simulink model "simulink_ros"  (R2022b)
settings: Solver=FixedStepAuto  StartTime=0.0  StopTime=10.0  FixedStep=0.01  RelTol=1e-3
libraries: robotlib x4
settings Model: Creator=pico  LastModifiedBy=pico

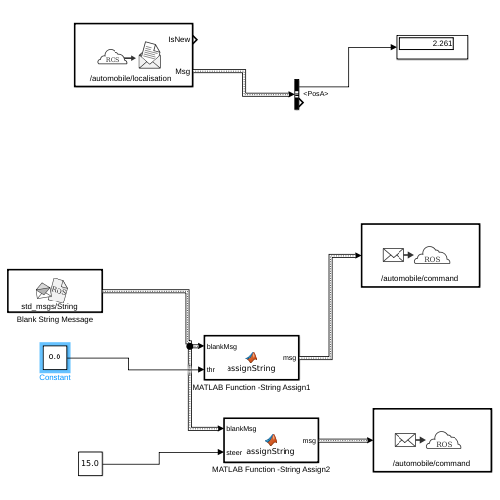
[thumbnail: Simulink's stored preview of the top-level diagram]
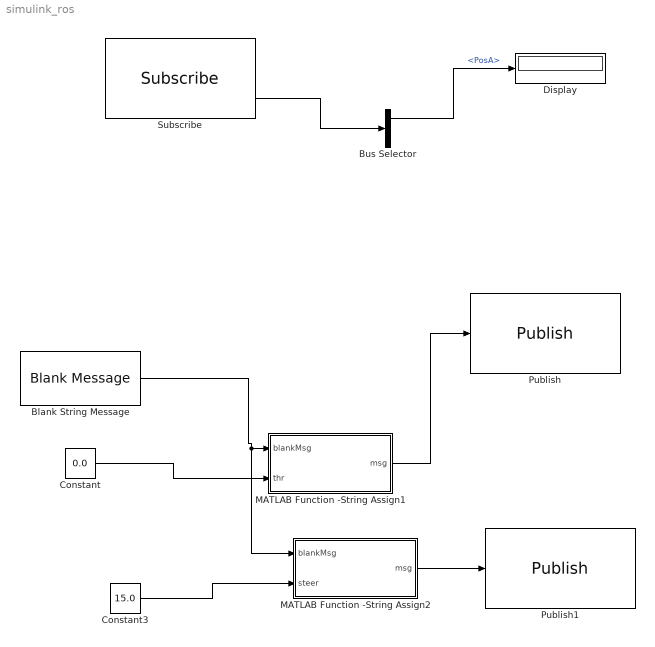
== system simulink_ros ==
  Blank String Message : robotlib/Blank Message  messageClass=Message  entityType=std_msgs/String  messageType=std_msgs/String  SampleTime=inf  legacyBusStruct=off
  Bus Selector : BusSelector  OutputSignals=PosA,PosB
  Constant : Constant  Value=0.0
  Constant3 : Constant  Value=15.0
  Display : Display
  MATLAB Function -String Assign1 : MATLAB Function  TreatAsAtomicUnit=on
  MATLAB Function -String Assign2 : MATLAB Function  TreatAsAtomicUnit=on
  Publish : robotlib/Publish  topicSource=Select from ROS network  topic=/automobile/command  messageType=std_msgs/String  legacyBusStruct=off  messageQueueLength=1
      settings: LibrarySourceBlock=roslib/ROS/Publish
  Publish1 : robotlib/Publish  topicSource=Select from ROS network  topic=/automobile/command  messageType=std_msgs/String  legacyBusStruct=off  messageQueueLength=1
      settings: LibrarySourceBlock=roslib/ROS/Publish
  Subscribe : robotlib/Subscribe  topicSource=Select from ROS network  topic=/automobile/localisation  messageType=utils/localisation  SampleTime=-1  legacyBusStruct=off  messageQueueLength=1
      settings: LibrarySourceBlock=roslib/ROS/Subscribe
  wires:
  Subscribe/2 -> Bus Selector/1
  Bus Selector/1 -> Display/1  "<PosA>"
  Blank String Message/1 -> MATLAB Function -String Assign2/1(blankMsg), MATLAB Function -String Assign1/1(blankMsg)
  MATLAB Function -String Assign1/1(msg) -> Publish/1
  Constant/1 -> MATLAB Function -String Assign1/2(thr)
  MATLAB Function -String Assign2/1(msg) -> Publish1/1
  Constant3/1 -> MATLAB Function -String Assign2/2(steer)

== matlab function simulink_ros/MATLAB Function -String Assign2 ==
  data: blankMsg input; msg output Bus: SL_Bus_simulink_ros_std_msgs_String; steer input
function msg = assignString(blankMsg,steer)
% assignString - Assign a string in a ROS message
%
% MSG = assignString(blankMsg) assigns a known string value to a 
%  string field in a ROS message, and outputs the updated ROS message.
%
%  blankMsg (input): A bus for a 'std_msgs/String' message. This is 
%      used to initialize the output. 
%  msg (output): A bus for a 'std_msgs/String' message, with the Data 
%      field set to a string.

%   Copyright 2015 The MathWorks, Inc.
%#codegen

% Note: The datatype of 'msg' has been explicitly set to the appropriate 
% Simulink bus type ("Bus: SL_Bus_robotROSMessageUsageExample_std_msgs_String"). 
%
% If the model name is changed, the datatype needs to be changed as well:
%   1) Click "Edit Data" in the Editor toolstrip to open "Ports and Data Manager"
%   2) Select "msg". From the "Type" dropdown, select "--- Refresh data types ---"
%   3) Set datatype to "Bus: SL_Bus_<modelname>_std_msgs_String"
    
% stringToAssign = 'information';
steer_string = sprintf('%.1f',steer);
% "{\"action\": \"1\", \"speed\": -0.1}"
stringToAssign = ['{"action": "2", "steerAngle": ',steer_string,'}'];%['action\', '1', 'speed',u];

msg = blankMsg;

% msg (std_msgs/String) consists of
%           Data : array of type uint8
%   Data_SL_Info : struct with fields CurrentLength, ReceivedLength
strLength = length(stringToAssign);
msg.Data(1:strLength) = uint8(stringToAssign);
msg.Data_SL_Info.CurrentLength = uint32(strLength);

== matlab function simulink_ros/MATLAB Function -String Assign1 ==
  data: blankMsg input; msg output Bus: SL_Bus_simulink_ros_std_msgs_String; thr input
function msg = assignString(blankMsg,thr)
% assignString - Assign a string in a ROS message
%
% MSG = assignString(blankMsg) assigns a known string value to a 
%  string field in a ROS message, and outputs the updated ROS message.
%
%  blankMsg (input): A bus for a 'std_msgs/String' message. This is 
%      used to initialize the output. 
%  msg (output): A bus for a 'std_msgs/String' message, with the Data 
%      field set to a string.

%   Copyright 2015 The MathWorks, Inc.
%#codegen

% Note: The datatype of 'msg' has been explicitly set to the appropriate 
% Simulink bus type ("Bus: SL_Bus_robotROSMessageUsageExample_std_msgs_String"). 
%
% If the model name is changed, the datatype needs to be changed as well:
%   1) Click "Edit Data" in the Editor toolstrip to open "Ports and Data Manager"
%   2) Select "msg". From the "Type" dropdown, select "--- Refresh data types ---"
%   3) Set datatype to "Bus: SL_Bus_<modelname>_std_msgs_String"
    
thr_string = sprintf('%.1f',thr);
% "{\"action\": \"1\", \"speed\": -0.1}"
stringToAssign = ['{"action": "1", "speed": ',thr_string,'}'];%['action\', '1', 'speed',u];

msg = blankMsg;

% msg (std_msgs/String) consists of
%           Data : array of type uint8
%   Data_SL_Info : struct with fields CurrentLength, ReceivedLength
strLength = length(stringToAssign);
msg.Data(1:strLength) = uint8(stringToAssign);
msg.Data_SL_Info.CurrentLength = uint32(strLength);
